simulink model "prueba"  (R2014a)
settings: Solver=ode8  StartTime=0.0  StopTime=inf  FixedStep=0.1  RelTol=1e-3
libraries: simulink x2, dspsrcs4 x1
settings Model: SimulationMode=external  PauseTimes=1  SnapshotBufferSize=1  SnapshotInterval=1  Creator=Jorge Luis Silva C  LastModifiedBy=Jorge Luis Silva C
settings HardwareCC: ProdIntDivRoundTo=Zero  ProdEndianess=LittleEndian  ProdHWDeviceType=Generic->32-bit x86 compatible
settings RTWCC: SystemTargetFile=rtwin.tlc  TemplateMakefile=rtwin.tmf  Description=Real-Time Windows Target  ProcessScript=rtwin_make_rtw_hook  RTWCompilerOptimization=On
settings CodeAppCC: MaxIdLength=95
settings RTWinTargetCC: TargetLibSuffix=_rtwin.lib  TargetPreCompLibLocation=C:\Program Files\MATLAB\R2014a\toolbox\rtw\targets\rtwin\lib\win64

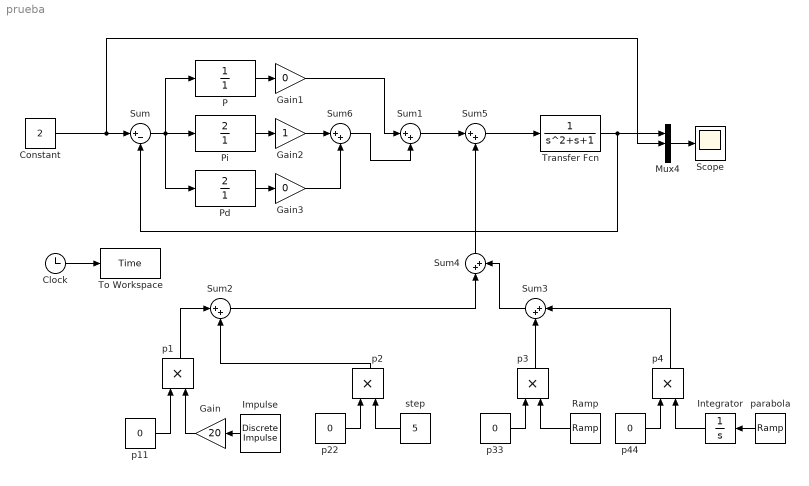
== system prueba ==
  " Impulse" : dspsrcs4/Discrete  Impulse  Delay=50  SampleTime=0.1  FrameSample=1  dataType=double  isSigned=on  wordLen=16  udDataType=sfix(16)  fracBitsMode=Best precision  numFracBits=15  OutDataTypeStr=double  LastOutDataTypeStr=double
  Clock : Clock
  Constant : Constant  Value=2
  Gain : Gain  Gain=20
  Gain1 : Gain  Gain=0
  Gain2 : Gain
  Gain3 : Gain  Gain=0
  Integrator : Integrator
  Mux4 : Mux  Inputs=3
      settings: DisplayOption=signals
  P : TransferFcn  Denominator=[1]
  Pd : TransferFcn  Numerator=[2]  Denominator=[1]
  Pi : TransferFcn  Numerator=[2]  Denominator=[1]
  Ramp : simulink/Sources/Ramp  slope=1  start=0  X0=0
  Scope : Scope
      settings: YMin=-150  YMax=950
  Sum : Sum  Inputs=|+-
  Sum{1..6} (6 alike) : Sum  Inputs=|++
  To Workspace : ToWorkspace  VariableName=Time  SaveFormat=Timeseries  SampleTime=-1
  Transfer Fcn : TransferFcn  Denominator=[1 1 1]
  p{1..4} (4 alike) : Product
  p{11,22,33,44} (4 alike) : Constant  Value=0
  parabola : simulink/Sources/Ramp  slope=1  start=0  X0=0
  step : Constant  Value=5
  wires:
  Sum/1 -> P/1, Pd/1, Pi/1
  Mux4/1 -> Scope/1
  Transfer Fcn/1 -> Mux4/1, Sum/2
  p22/1 -> p2/1
  p1/1 -> Sum2/1
  p2/1 -> Sum2/2
  step/1 -> p2/2
  p44/1 -> p4/1
  p4/1 -> Sum3/1
  Integrator/1 -> p4/2
  p11/1 -> p1/1
  " Impulse"/1 -> Gain/1
  Gain/1 -> p1/2
  p33/1 -> p3/1
  p3/1 -> Sum3/2
  Ramp/1 -> p3/2
  Sum2/1 -> Sum4/1
  Sum3/1 -> Sum4/2
  parabola/1 -> Integrator/1
  P/1 -> Gain1/1
  Pi/1 -> Gain2/1
  Pd/1 -> Gain3/1
  Constant/1 -> Mux4/2, Sum/1
  Gain2/1 -> Sum6/1
  Gain3/1 -> Sum6/2
  Sum6/1 -> Sum1/2
  Gain1/1 -> Sum1/1
  Sum1/1 -> Sum5/1
  Sum5/1 -> Transfer Fcn/1
  Sum4/1 -> Sum5/2
  Clock/1 -> To Workspace/1
